simulink model "step_i_add_zeros"  (R2021a)
settings: Solver=VariableStepAuto  StartTime=0.0  StopTime=10.0  RelTol=1e-3
values from neighbouring files (symbols this model uses):
  b = 20000    [matlab_code.m]
  j = 600000    [matlab_code.m]
  k = 2000    [matlab_code.m]
settings Model: Creator=dyab  LastModifiedBy=dyab

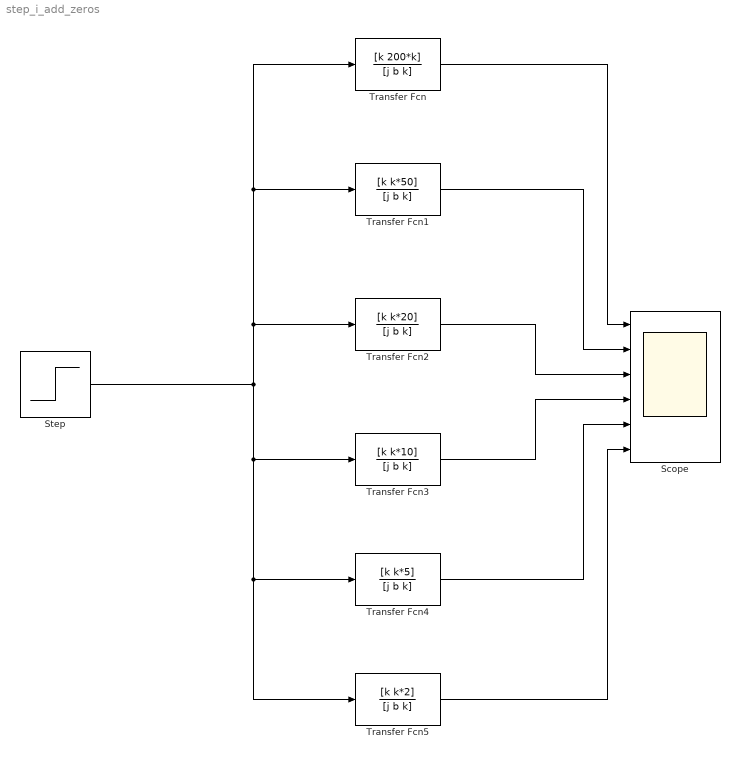
== system step_i_add_zeros ==
  Scope : Scope  NumInputPorts=6
  Step : Step  SampleTime=0
  Transfer Fcn : TransferFcn  Numerator=[k 200*k]  Denominator=[j b k]
  Transfer Fcn1 : TransferFcn  Numerator=[k k*50]  Denominator=[j b k]
  Transfer Fcn2 : TransferFcn  Numerator=[k k*20]  Denominator=[j b k]
  Transfer Fcn3 : TransferFcn  Numerator=[k k*10]  Denominator=[j b k]
  Transfer Fcn4 : TransferFcn  Numerator=[k k*5]  Denominator=[j b k]
  Transfer Fcn5 : TransferFcn  Numerator=[k k*2]  Denominator=[j b k]
  wires:
  Transfer Fcn2/1 -> Scope/3
  Transfer Fcn3/1 -> Scope/4
  Transfer Fcn4/1 -> Scope/5
  Transfer Fcn5/1 -> Scope/6
  Transfer Fcn1/1 -> Scope/2
  Transfer Fcn/1 -> Scope/1
  Step/1 -> Transfer Fcn5/1, Transfer Fcn4/1, Transfer Fcn3/1, Transfer Fcn/1, Transfer Fcn1/1, Transfer Fcn2/1
